simulink model "Model_Initialize"  (R2025b)
settings: Solver=FixedStepAuto  StartTime=0.0  StopTime=100  FixedStep=.05  RelTol=1e-3
values from neighbouring files (symbols this model uses):
  Cbv0 = Cb2*C21*C1v    [Euler_Kinematical_Equations.m]
  phi0 = 0    [Euler_Kinematical_Equations.m]
  psi0 = 0    [Euler_Kinematical_Equations.m]
  q0 = angle2quat(psi0,theta0,phi0)    [Euler_Kinematical_Equations.m]
  theta0 = 0.0059    [Euler_Kinematical_Equations.m]
settings Model: Creator=nuris  LastModifiedBy=nuris

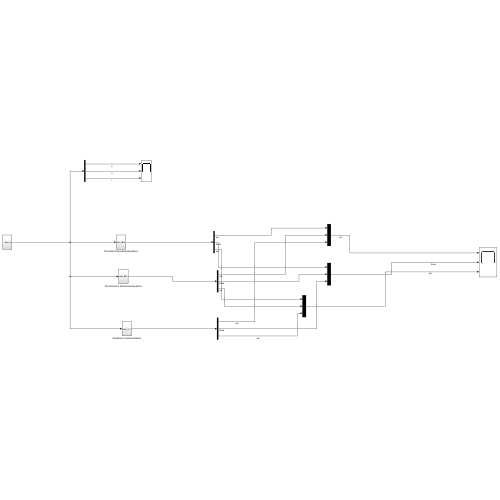
[thumbnail: Simulink's stored preview of the top-level diagram]
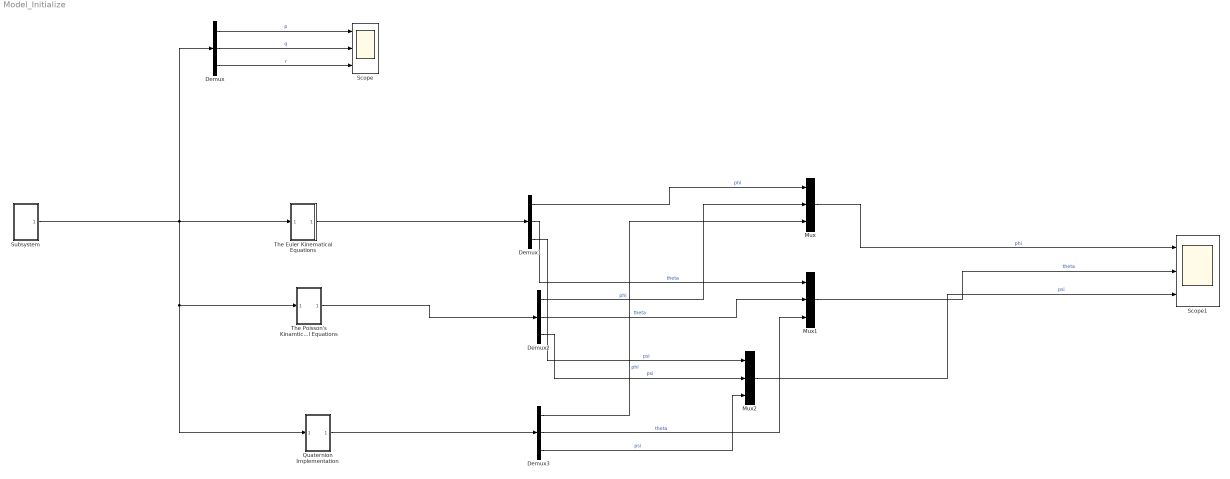
== system Model_Initialize ==
  Demux{,1..3} (4 alike) : Demux  Outputs=3
  Mux : Mux  Inputs=3
  Mux1 : Mux  Inputs=3
  Mux2 : Mux  Inputs=3
  Quaternion Implementation : Subsystem
  Scope : Scope  NumInputPorts=3
      settings: ActiveDisplayYMinimum=-0.18408759353078635  ActiveDisplayYMaximum=0.20426118531120285
  Scope1 : Scope  NumInputPorts=3
      settings: ActiveDisplayYMinimum=-0.13336457236381291  ActiveDisplayYMaximum=1.2002811512743166
  Subsystem : Subsystem
  The Euler Kinematical Equations : Subsystem
  The Poisson's Kinamtical Equations : Subsystem
  wires:
  Subsystem/1(wbv_b) -> Quaternion Implementation/1(wbv_b), The Poisson's Kinamtical Equations/1(wbv_b), The Euler Kinematical Equations/1(wbv_b), Demux/1
  Demux/1 -> Scope/1  "p"
  Demux/2 -> Scope/2  "q"
  Demux/3 -> Scope/3  "r"
  The Euler Kinematical Equations/1(Phi) -> Demux1/1
  The Poisson's Kinamtical Equations/1(Phi) -> Demux2/1
  Demux1/1 -> Mux/1  "phi"
  Demux2/1 -> Mux/2  "phi"
  Mux/1 -> Scope1/1  "phi"
  Demux1/2 -> Mux1/1  "theta"
  Mux1/1 -> Scope1/2  "theta"
  Demux1/3 -> Mux2/1  "psi"
  Demux2/3 -> Mux2/2  "psi"
  Mux2/1 -> Scope1/3  "psi"
  Demux3/1 -> Mux/3  "phi"
  Demux3/3 -> Mux2/3  "psi"
  Quaternion Implementation/1(Out1) -> Demux3/1
  Demux2/2 -> Mux1/2  "theta"
  Demux3/2 -> Mux1/3  "theta"

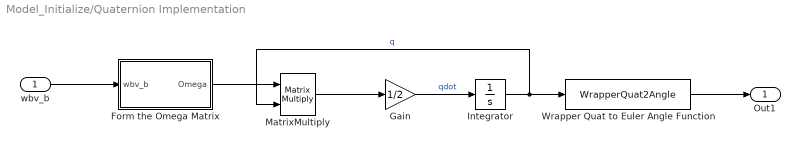
== system Model_Initialize/Quaternion Implementation ==
  wbv_b : Inport
  Form the Omega Matrix : MATLAB Function  TreatAsAtomicUnit=on
  Gain : Gain  Gain=1/2
  Integrator : Integrator  InitialCondition=q0
  MatrixMultiply : Product  Multiplication=Matrix(*)
  Wrapper Quat to Euler Angle Function : MATLABFcn  MATLABFcn=WrapperQuat2Angle
  Out1 : Outport
  wires:
  wbv_b/1 -> Form the Omega Matrix/1(wbv_b)
  Form the Omega Matrix/1(Omega) -> MatrixMultiply/1
  MatrixMultiply/1 -> Gain/1
  Gain/1 -> Integrator/1  "qdot"
  Integrator/1 -> Wrapper Quat to Euler Angle Function/1, MatrixMultiply/2  "q"
  Wrapper Quat to Euler Angle Function/1 -> Out1/1

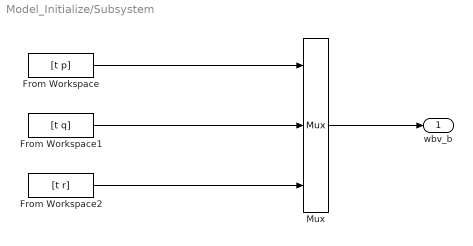
== system Model_Initialize/Subsystem ==
  From Workspace : FromWorkspace  VariableName=[t p]
  From Workspace1 : FromWorkspace  VariableName=[t q]
  From Workspace2 : FromWorkspace  VariableName=[t r]
  Mux : Mux  Inputs=3
  wbv_b : Outport
  wires:
  From Workspace/1 -> Mux/1
  From Workspace1/1 -> Mux/2
  From Workspace2/1 -> Mux/3
  Mux/1 -> wbv_b/1

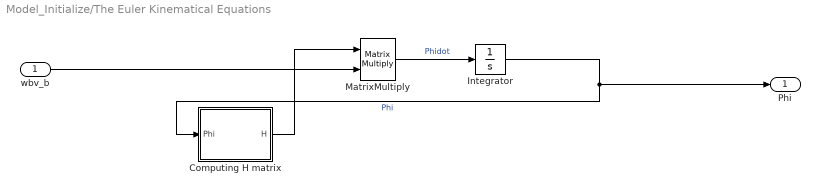
== system Model_Initialize/The Euler Kinematical Equations ==
  wbv_b : Inport
  Computing H matrix : MATLAB Function  TreatAsAtomicUnit=on
  Integrator : Integrator  InitialCondition=[phi0;theta0;psi0]
  MatrixMultiply : Product  Multiplication=Matrix(*)
  Phi : Outport
  wires:
  MatrixMultiply/1 -> Integrator/1  "Phidot"
  Integrator/1 -> Phi/1, Computing H matrix/1(Phi)  "Phi"
  Computing H matrix/1(H) -> MatrixMultiply/1
  wbv_b/1 -> MatrixMultiply/2

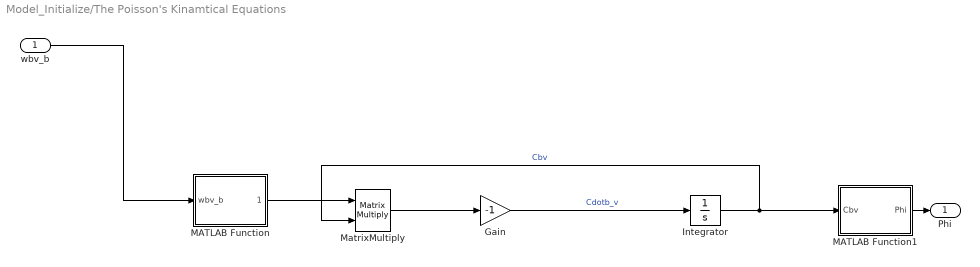
== system Model_Initialize/The Poisson's Kinamtical Equations ==
  wbv_b : Inport
  Gain : Gain  Gain=-1
  Integrator : Integrator  InitialCondition=Cbv0
  MATLAB Function : MATLAB Function  TreatAsAtomicUnit=on
  MATLAB Function1 : MATLAB Function  TreatAsAtomicUnit=on
  MatrixMultiply : Product  Multiplication=Matrix(*)
  Phi : Outport
  wires:
  Integrator/1 -> MATLAB Function1/1(Cbv), MatrixMultiply/2  "Cbv"
  MATLAB Function/1(Omega_bv_b) -> MatrixMultiply/1
  MatrixMultiply/1 -> Gain/1
  Gain/1 -> Integrator/1  "Cdotb_v"
  wbv_b/1 -> MATLAB Function/1(wbv_b)
  MATLAB Function1/1(Phi) -> Phi/1

== matlab function Model_Initialize/The Poisson's Kinamtical Equations/MATLAB Function ==
  data: wbv_b input; Omega_bv_b output
function Omega_bv_b = fcn(wbv_b)



p = wbv_b(1);
q = wbv_b(2);
r = wbv_b(3);

Omega_bv_b = [0 -r q;
    r 0 -p;
    -q p 0];

== matlab function Model_Initialize/The Euler Kinematical Equations/Computing H matrix ==
  data: H output; Phi input
function H = fcn(Phi)

%Unpack Phi
phi     = Phi(1);
theta   = Phi(2);
psi     = Phi(3);

%Input the H matrix
H = [1 tan(theta)*sin(phi) tan(theta)*cos(phi);
    0 cos(phi) -sin(phi);
    0 sin(phi)/cos(theta) cos(phi)/cos(theta)];

== matlab function Model_Initialize/The Poisson's Kinamtical Equations/MATLAB Function1 ==
  data: Cbv input; Phi output
function Phi = fcn(Cbv)

c11 = Cbv(1,1);
c13 = Cbv(1,3);
c12 = Cbv(1,2);
c23 = Cbv(2,3);
c33 = Cbv(3,3);

phi = atan2(c23,c33);
theta = -asin(c13);
psi2 = atan2(c12,c11); % avoid problem with function called psi


Phi = [phi;theta;psi2];

== matlab function Model_Initialize/Quaternion Implementation/Form the Omega Matrix ==
  data: wbv_b input; Omega output
function Omega = fcn(wbv_b)

wx = wbv_b(1);
wy = wbv_b(2);
wz = wbv_b(3);

Omega = [0 -wx -wy -wz;
        wx 0 wz -wy;
        wy -wz 0 wx;
        wz wy -wx 0];
